simulink model "Generator_Boeing_project"  (R2019a)
settings: Solver=VariableStepAuto  StartTime=0.0  StopTime=10.0  RelTol=1e-3
values from neighbouring files (symbols this model uses):
  Lls = 4*2.822e-6    (= 1.1288e-05)    [Generator_parameters.m]
  Lmd = 4*164.571e-6    (= 0.000658284)    [Generator_parameters.m]
  Lmq = 4*125.772e-6    (= 0.000503088)    [Generator_parameters.m]
  Lpfd = 4.9*6e-6    (= 2.94e-05)    [Generator_parameters.m]
  Lpkd = 16*9.093e-6    (= 0.000145488)    [Generator_parameters.m]
  Lpkq = 16*3.175e-6    (= 5.08e-05)    [Generator_parameters.m]
  Nfds_gen = 25    [Generator_parameters.m]
  Ra = 4*2.794e-3    (= 0.011176)    [Generator_parameters.m]
  Rpfd = 4*634.998e-6    (= 0.002539992)    [Generator_parameters.m]
  Rpkd = 8*11.72e-3    (= 0.09376)    [Generator_parameters.m]
  Rpkq = 8*3.712e-3    (= 0.029696)    [Generator_parameters.m]
undefined symbols (not defined in the file or in its folder): ts
settings Model: Creator=Dominion  LastModifiedBy=Dominion

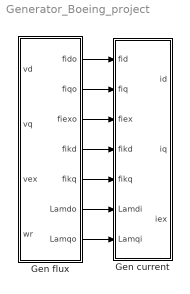
== system Generator_Boeing_project ==
  Gen current : Subsystem
  Gen flux : Subsystem
  wires:
  Gen flux/4(fikd) -> Gen current/4(fikd)
  Gen flux/5(fikq) -> Gen current/5(fikq)
  Gen flux/3(fiexo) -> Gen current/3(fiex)
  ? -> Gen flux/1(vd)
  Gen flux/7(Lamqo) -> Gen current/7(Lamqi)
  ? -> Gen flux/2(vq)
  Gen flux/2(fiqo) -> Gen current/2(fiq)
  Gen flux/6(Lamdo) -> Gen current/6(Lamdi)
  ? -> Gen flux/4(wr)
  Gen flux/1(fido) -> Gen current/1(fid)
  ? -> Gen flux/3(vex)

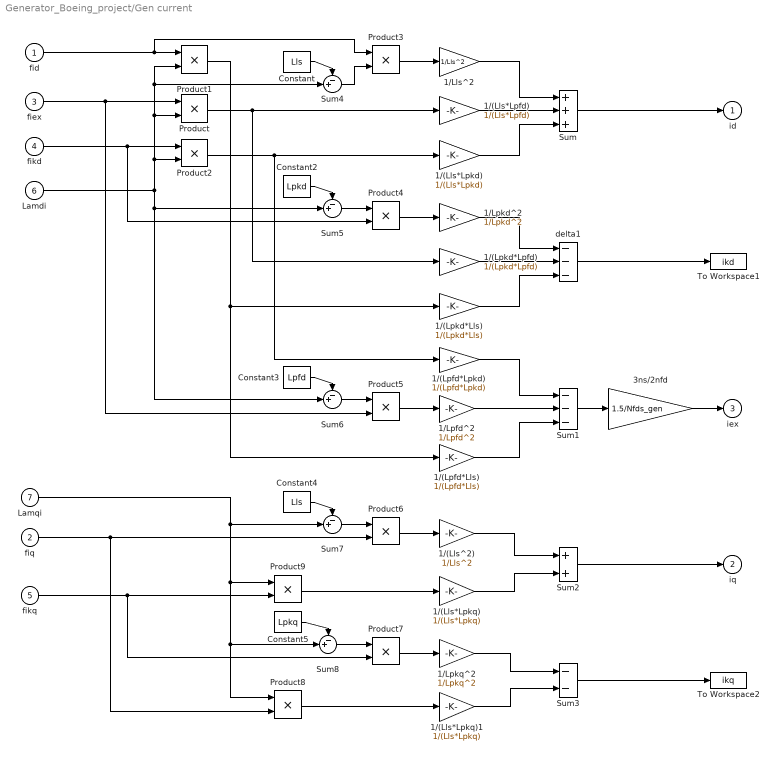
== system Generator_Boeing_project/Gen current ==
  fid : Inport
  fiq : Inport  Port=2
  fiex : Inport  Port=3
  fikd : Inport  Port=4
  fikq : Inport  Port=5
  Lamdi : Inport  Port=6
  Lamqi : Inport  Port=7
  1/(Lls*Lpfd) : Gain  Gain=1/(Lls*Lpfd)  SaturateOnIntegerOverflow=on  OutDataTypeStr=Inherit: Same as input  ParamDataTypeStr=Inherit: Same as input
  1/(Lls*Lpkd) : Gain  Gain=1/(Lls*Lpkd)  SaturateOnIntegerOverflow=on  OutDataTypeStr=Inherit: Same as input  ParamDataTypeStr=Inherit: Same as input
  1/(Lls*Lpkq) : Gain  Gain=1/(Lls*Lpkq)  SaturateOnIntegerOverflow=on  OutDataTypeStr=Inherit: Same as input  ParamDataTypeStr=Inherit: Same as input
  1/(Lls*Lpkq)1 : Gain  Gain=1/(Lls*Lpkq)  SaturateOnIntegerOverflow=on  OutDataTypeStr=Inherit: Same as input  ParamDataTypeStr=Inherit: Same as input
  1/(Lls^2) : Gain  Gain=1/Lls^2  SaturateOnIntegerOverflow=on  OutDataTypeStr=Inherit: Same as input  ParamDataTypeStr=Inherit: Same as input
  1/(Lpfd*Lls) : Gain  Gain=1/(Lpfd*Lls)  SaturateOnIntegerOverflow=on  OutDataTypeStr=Inherit: Same as input  ParamDataTypeStr=Inherit: Same as input
  1/(Lpfd*Lpkd) : Gain  Gain=1/(Lpfd*Lpkd)  SaturateOnIntegerOverflow=on  OutDataTypeStr=Inherit: Same as input  ParamDataTypeStr=Inherit: Same as input
  1/(Lpkd*Lls) : Gain  Gain=1/(Lpkd*Lls)  SaturateOnIntegerOverflow=on  OutDataTypeStr=Inherit: Same as input  ParamDataTypeStr=Inherit: Same as input
  1/(Lpkd*Lpfd) : Gain  Gain=1/(Lpkd*Lpfd)  SaturateOnIntegerOverflow=on  OutDataTypeStr=Inherit: Same as input  ParamDataTypeStr=Inherit: Same as input
  1/Lls^2 : Gain  Gain=1/Lls^2  SaturateOnIntegerOverflow=on  OutDataTypeStr=Inherit: Same as input  ParamDataTypeStr=Inherit: Same as input
  1/Lpfd^2 : Gain  Gain=1/Lpfd^2  SaturateOnIntegerOverflow=on  OutDataTypeStr=Inherit: Same as input  ParamDataTypeStr=Inherit: Same as input
  1/Lpkd^2 : Gain  Gain=1/Lpkd^2  SaturateOnIntegerOverflow=on  OutDataTypeStr=Inherit: Same as input  ParamDataTypeStr=Inherit: Same as input
  1/Lpkq^2 : Gain  Gain=1/Lpkq^2  SaturateOnIntegerOverflow=on  OutDataTypeStr=Inherit: Same as input  ParamDataTypeStr=Inherit: Same as input
  3ns/2nfd : Gain  Gain=1.5/Nfds_gen  SaturateOnIntegerOverflow=on  OutDataTypeStr=Inherit: Same as input  ParamDataTypeStr=Inherit: Same as input
  Constant : Constant  Value=Lls
  Constant2 : Constant  Value=Lpkd
  Constant3 : Constant  Value=Lpfd
  Constant4 : Constant  Value=Lls
  Constant5 : Constant  Value=Lpkq
  Product{,1..9} (10 alike) : Product  RndMeth=Zero
  Sum : Sum  Inputs=+++  SaturateOnIntegerOverflow=on  InputSameDT=on  OutDataTypeStr=Inherit: Same as first input
  Sum1 : Sum  Inputs=---  SaturateOnIntegerOverflow=on  InputSameDT=on  OutDataTypeStr=Inherit: Same as first input
  Sum2 : Sum  SaturateOnIntegerOverflow=on  InputSameDT=on  OutDataTypeStr=Inherit: Same as first input
  Sum3 : Sum  Inputs=--  SaturateOnIntegerOverflow=on  InputSameDT=on  OutDataTypeStr=Inherit: Same as first input
  Sum{4..8} (5 alike) : Sum  Inputs=-+|
  To Workspace1 : ToWorkspace  VariableName=ikd  SampleTime=ts
  To Workspace2 : ToWorkspace  VariableName=ikq  SampleTime=ts
  delta1 : Sum  Inputs=---  SaturateOnIntegerOverflow=on  InputSameDT=on  OutDataTypeStr=Inherit: Same as first input
  id : Outport
  iq : Outport  Port=2
  iex : Outport  Port=3
  wires:
  fiq/1 -> Product6/2, Product8/2
  fid/1 -> Product1/1, Product3/1
  Sum/1 -> id/1
  Sum1/1 -> 3ns/2nfd/1
  Sum2/1 -> iq/1
  1/(Lls*Lpkd)/1 -> Sum/3
  delta1/1 -> To Workspace1/1
  1/(Lpkd*Lpfd)/1 -> delta1/2
  1/Lpkd^2/1 -> delta1/1
  1/(Lpfd*Lpkd)/1 -> Sum1/1
  1/(Lls^2)/1 -> Sum2/1
  1/(Lls*Lpkq)/1 -> Sum2/2
  1/Lls^2/1 -> Sum/1
  fiex/1 -> Product/1, Product5/2
  1/(Lls*Lpfd)/1 -> Sum/2
  fikd/1 -> Product2/1, Product4/2
  1/(Lpkd*Lls)/1 -> delta1/3
  1/Lpfd^2/1 -> Sum1/2
  1/(Lpfd*Lls)/1 -> Sum1/3
  fikq/1 -> Product7/2, Product9/2
  Sum3/1 -> To Workspace2/1
  1/Lpkq^2/1 -> Sum3/1
  1/(Lls*Lpkq)1/1 -> Sum3/2
  Product/1 -> 1/(Lls*Lpfd)/1, 1/(Lpkd*Lpfd)/1
  Lamdi/1 -> Product/2, Product1/2, Sum4/2, Product2/2, Sum5/2, Sum6/2
  Product1/1 -> 1/(Lpkd*Lls)/1, 1/(Lpfd*Lls)/1
  Product2/1 -> 1/(Lls*Lpkd)/1, 1/(Lpfd*Lpkd)/1
  Product3/1 -> 1/Lls^2/1
  Constant/1 -> Sum4/1
  Sum4/1 -> Product3/2
  Product4/1 -> 1/Lpkd^2/1
  Sum5/1 -> Product4/1
  Constant2/1 -> Sum5/1
  Constant3/1 -> Sum6/1
  Product5/1 -> 1/Lpfd^2/1
  Sum6/1 -> Product5/1
  Product6/1 -> 1/(Lls^2)/1
  Lamqi/1 -> Sum7/2, Sum8/2, Product8/1, Product9/1
  Constant4/1 -> Sum7/1
  Sum7/1 -> Product6/1
  Constant5/1 -> Sum8/1
  Product7/1 -> 1/Lpkq^2/1
  Sum8/1 -> Product7/1
  Product8/1 -> 1/(Lls*Lpkq)1/1
  Product9/1 -> 1/(Lls*Lpkq)/1
  3ns/2nfd/1 -> iex/1

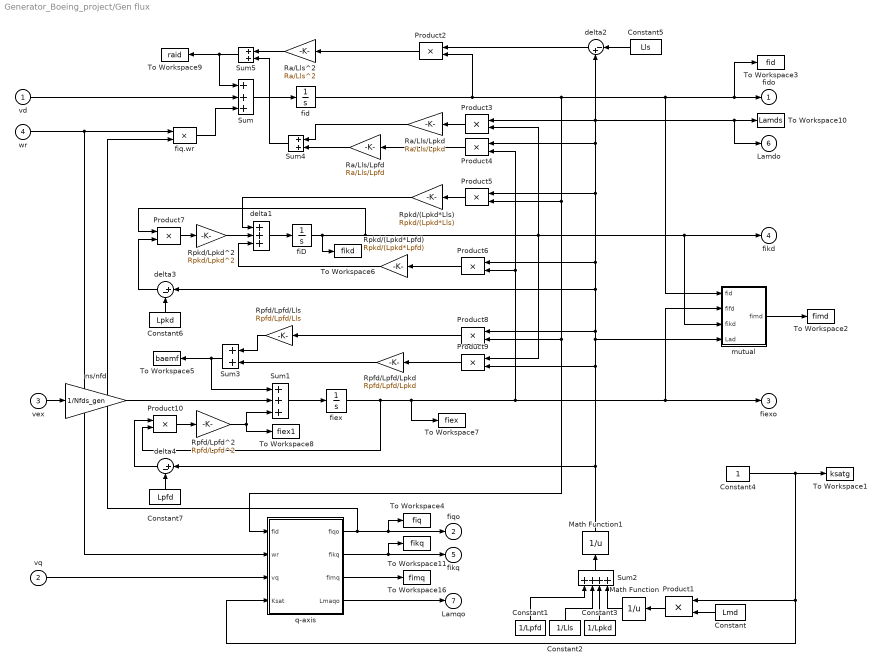
== system Generator_Boeing_project/Gen flux ==
  vd : Inport
  vq : Inport  Port=2
  vex : Inport  Port=3
  wr : Inport  Port=4
  Constant : Constant  Value=Lmd
  Constant1 : Constant  Value=1/Lpfd
  Constant2 : Constant  Value=1/Lls
  Constant3 : Constant  Value=1/Lpkd
  Constant4 : Constant
  Constant5 : Constant  Value=Lls
  Constant6 : Constant  Value=Lpkd
  Constant7 : Constant  Value=Lpfd
  Math Function : Math  Operator=reciprocal  SaturateOnIntegerOverflow=on
  Math Function1 : Math  Operator=reciprocal  SaturateOnIntegerOverflow=on
  Product{1..10} (10 alike) : Product  SaturateOnIntegerOverflow=on  OutDataTypeStr=Inherit: Same as first input
  Ra/Lls/Lpfd : Gain  Gain=Ra/Lls/Lpfd  SaturateOnIntegerOverflow=on  OutDataTypeStr=Inherit: Same as input  ParamDataTypeStr=Inherit: Same as input
  Ra/Lls/Lpkd : Gain  Gain=Ra/Lls/Lpkd  SaturateOnIntegerOverflow=on  OutDataTypeStr=Inherit: Same as input  ParamDataTypeStr=Inherit: Same as input
  Ra/Lls^2 : Gain  Gain=Ra/Lls^2  SaturateOnIntegerOverflow=on  OutDataTypeStr=Inherit: Same as input  ParamDataTypeStr=Inherit: Same as input
  Rpfd/Lpfd/Lls : Gain  Gain=Rpfd/Lpfd/Lls  SaturateOnIntegerOverflow=on  OutDataTypeStr=Inherit: Same as input  ParamDataTypeStr=Inherit: Same as input
  Rpfd/Lpfd/Lpkd : Gain  Gain=Rpfd/Lpfd/Lpkd  SaturateOnIntegerOverflow=on  OutDataTypeStr=Inherit: Same as input  ParamDataTypeStr=Inherit: Same as input
  Rpfd/Lpfd^2 : Gain  Gain=Rpfd/Lpfd^2  SaturateOnIntegerOverflow=on  OutDataTypeStr=Inherit: Same as input  ParamDataTypeStr=Inherit: Same as input
  Rpkd/(Lpkd*Lls) : Gain  Gain=Rpkd/(Lpkd*Lls)  SaturateOnIntegerOverflow=on  OutDataTypeStr=Inherit: Same as input  ParamDataTypeStr=Inherit: Same as input
  Rpkd/(Lpkd*Lpfd) : Gain  Gain=Rpkd/(Lpkd*Lpfd)  SaturateOnIntegerOverflow=on  OutDataTypeStr=Inherit: Same as input  ParamDataTypeStr=Inherit: Same as input
  Rpkd/Lpkd^2 : Gain  Gain=Rpkd/Lpkd^2  SaturateOnIntegerOverflow=on  OutDataTypeStr=Inherit: Same as input  ParamDataTypeStr=Inherit: Same as input
  Sum : Sum  Inputs=+++  SaturateOnIntegerOverflow=on  InputSameDT=on  OutDataTypeStr=Inherit: Same as first input
  Sum1 : Sum  Inputs=+++  SaturateOnIntegerOverflow=on  InputSameDT=on  OutDataTypeStr=Inherit: Same as first input
  Sum2 : Sum  Inputs=++++  SaturateOnIntegerOverflow=on  InputSameDT=on  OutDataTypeStr=Inherit: Same as first input
  Sum3 : Sum  SaturateOnIntegerOverflow=on  InputSameDT=on  OutDataTypeStr=Inherit: Same as first input
  Sum4 : Sum  SaturateOnIntegerOverflow=on  InputSameDT=on  OutDataTypeStr=Inherit: Same as first input
  Sum5 : Sum  SaturateOnIntegerOverflow=on  InputSameDT=on  OutDataTypeStr=Inherit: Same as first input
  To Workspace1 : ToWorkspace  VariableName=ksatg  SampleTime=ts
  To Workspace10 : ToWorkspace  VariableName=Lamds  SampleTime=ts
  To Workspace11 : ToWorkspace  VariableName=fikq  SampleTime=ts
  To Workspace16 : ToWorkspace  VariableName=fimq  SampleTime=ts
  To Workspace2 : ToWorkspace  VariableName=fimd  SampleTime=ts
  To Workspace3 : ToWorkspace  VariableName=fid  SampleTime=ts
  To Workspace4 : ToWorkspace  VariableName=fiq  SampleTime=ts
  To Workspace5 : ToWorkspace  VariableName=baemf  SampleTime=ts
  To Workspace6 : ToWorkspace  VariableName=fikd  SampleTime=ts
  To Workspace7 : ToWorkspace  VariableName=fiex  SampleTime=ts
  To Workspace8 : ToWorkspace  VariableName=fiex1  SampleTime=ts
  To Workspace9 : ToWorkspace  VariableName=raid  SampleTime=ts
  delta1 : Sum  Inputs=+++  SaturateOnIntegerOverflow=on  InputSameDT=on  OutDataTypeStr=Inherit: Same as first input
  delta2 : Sum  Inputs=|-+  SaturateOnIntegerOverflow=on  InputSameDT=on  OutDataTypeStr=Inherit: Same as first input
  delta3 : Sum  Inputs=|+-  SaturateOnIntegerOverflow=on  InputSameDT=on  OutDataTypeStr=Inherit: Same as first input
  delta4 : Sum  Inputs=|+-  SaturateOnIntegerOverflow=on  InputSameDT=on  OutDataTypeStr=Inherit: Same as first input
  fiD : Integrator
  fid : Integrator
  fiex : Integrator
  fiq.wr : Product  SaturateOnIntegerOverflow=on  InputSameDT=on  OutDataTypeStr=Inherit: Same as first input
  mutual : Subsystem
  ns/nfd : Gain  Gain=1/Nfds_gen  SaturateOnIntegerOverflow=on  OutDataTypeStr=Inherit: Same as input  ParamDataTypeStr=Inherit: Same as input
  q-axis : Subsystem
  fido : Outport
  fiqo : Outport  Port=2
  fiexo : Outport  Port=3
  fikd : Outport  Port=4
  fikq : Outport  Port=5
  Lamdo : Outport  Port=6
  Lamqo : Outport  Port=7
  wires:
  fid/1 -> Product5/2, q-axis/1(fid), Product8/2, mutual/1(fid), fido/1, To Workspace3/1, Product2/2
  vd/1 -> Sum/2
  Sum/1 -> fid/1
  Sum1/1 -> fiex/1
  fiq.wr/1 -> Sum/3
  fiex/1 -> Product10/2, Product4/2, Product6/2, fiexo/1, mutual/2(fifd), To Workspace7/1
  fiD/1 -> Product3/2, Product9/1, fikd/1, mutual/3(fikd), Product7/1, To Workspace6/1
  Product2/1 -> Ra/Lls^2/1
  Ra/Lls/Lpkd/1 -> Sum4/1
  Ra/Lls/Lpfd/1 -> Sum4/2
  delta1/1 -> fiD/1
  Rpkd/Lpkd^2/1 -> delta1/2
  Rpkd/(Lpkd*Lls)/1 -> delta1/1
  Rpkd/(Lpkd*Lpfd)/1 -> delta1/3
  vex/1 -> ns/nfd/1
  wr/1 -> fiq.wr/1, q-axis/2(wr)
  vq/1 -> q-axis/3(vq)
  q-axis/1(fiqo) -> fiq.wr/2, fiqo/1, To Workspace4/1
  q-axis/2(fikq) -> fikq/1, To Workspace11/1
  q-axis/3(fimq) -> To Workspace16/1
  Constant1/1 -> Sum2/1
  Constant2/1 -> Sum2/2
  Constant3/1 -> Sum2/3
  Math Function/1 -> Sum2/4
  Constant5/1 -> delta2/1
  Sum2/1 -> Math Function1/1
  delta2/1 -> Product2/1
  Product3/1 -> Ra/Lls/Lpkd/1
  Product4/1 -> Ra/Lls/Lpfd/1
  Product5/1 -> Rpkd/(Lpkd*Lls)/1
  Product6/1 -> Rpkd/(Lpkd*Lpfd)/1
  Constant6/1 -> delta3/2
  delta3/1 -> Product7/2
  Product7/1 -> Rpkd/Lpkd^2/1
  Product8/1 -> Rpfd/Lpfd/Lls/1
  Product9/1 -> Rpfd/Lpfd/Lpkd/1
  Constant7/1 -> delta4/2
  Product10/1 -> Rpfd/Lpfd^2/1
  delta4/1 -> Product10/1
  Math Function1/1 -> Product9/2, delta2/2, Product3/1, To Workspace10/1, Lamdo/1, Product4/1, Product5/1, Product6/1, delta3/1, Product8/1, mutual/4(Lad), delta4/1
  Constant/1 -> Product1/2
  Product1/1 -> Math Function/1
  mutual/1(fimd) -> To Workspace2/1
  Rpfd/Lpfd^2/1 -> Sum1/3, To Workspace8/1
  Rpfd/Lpfd/Lls/1 -> Sum3/1
  Rpfd/Lpfd/Lpkd/1 -> Sum3/2
  Sum3/1 -> Sum1/1, To Workspace5/1
  Ra/Lls^2/1 -> Sum5/1
  Sum4/1 -> Sum5/2
  Sum5/1 -> Sum/1, To Workspace9/1
  q-axis/4(Lmaqo) -> Lamqo/1
  ns/nfd/1 -> Sum1/2
  Constant4/1 -> To Workspace1/1, Product1/1, q-axis/4(Ksat)

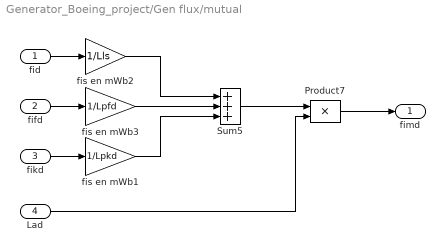
== system Generator_Boeing_project/Gen flux/mutual ==
  fid : Inport
  fifd : Inport  Port=2
  fikd : Inport  Port=3
  Lad : Inport  Port=4
  Product7 : Product  SaturateOnIntegerOverflow=on  OutDataTypeStr=Inherit: Same as first input
  Sum5 : Sum  Inputs=+++  SaturateOnIntegerOverflow=on  InputSameDT=on  OutDataTypeStr=Inherit: Same as first input
  fis en mWb1 : Gain  Gain=1/Lpkd  SaturateOnIntegerOverflow=on  OutDataTypeStr=Inherit: Same as input  ParamDataTypeStr=Inherit: Same as input
  fis en mWb2 : Gain  Gain=1/Lls  SaturateOnIntegerOverflow=on  OutDataTypeStr=Inherit: Same as input  ParamDataTypeStr=Inherit: Same as input
  fis en mWb3 : Gain  Gain=1/Lpfd  SaturateOnIntegerOverflow=on  OutDataTypeStr=Inherit: Same as input  ParamDataTypeStr=Inherit: Same as input
  fimd : Outport
  wires:
  fis en mWb1/1 -> Sum5/3
  fis en mWb3/1 -> Sum5/2
  fis en mWb2/1 -> Sum5/1
  fid/1 -> fis en mWb2/1
  fifd/1 -> fis en mWb3/1
  fikd/1 -> fis en mWb1/1
  Sum5/1 -> Product7/1
  Product7/1 -> fimd/1
  Lad/1 -> Product7/2

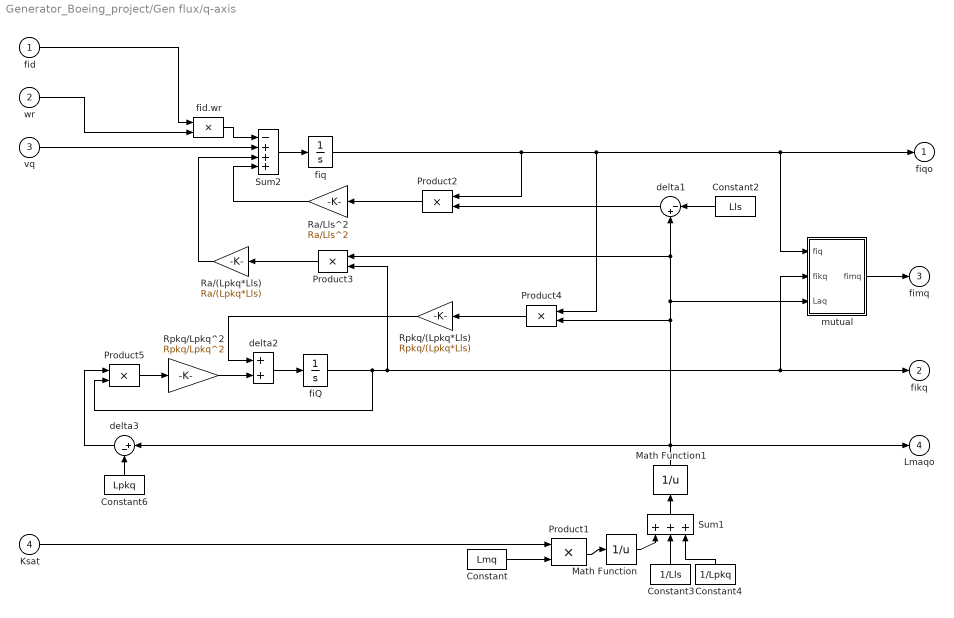
== system Generator_Boeing_project/Gen flux/q-axis ==
  fid : Inport
  wr : Inport  Port=2
  vq : Inport  Port=3
  Ksat : Inport  Port=4
  Constant : Constant  Value=Lmq
  Constant2 : Constant  Value=Lls
  Constant3 : Constant  Value=1/Lls
  Constant4 : Constant  Value=1/Lpkq
  Constant6 : Constant  Value=Lpkq
  Math Function : Math  Operator=reciprocal  SaturateOnIntegerOverflow=on
  Math Function1 : Math  Operator=reciprocal  SaturateOnIntegerOverflow=on
  Product{1..5} (5 alike) : Product  SaturateOnIntegerOverflow=on  OutDataTypeStr=Inherit: Same as first input
  Ra/(Lpkq*Lls) : Gain  Gain=Ra/(Lpkq*Lls)  SaturateOnIntegerOverflow=on  OutDataTypeStr=Inherit: Same as input  ParamDataTypeStr=Inherit: Same as input
  Ra/Lls^2 : Gain  Gain=Ra/Lls^2  SaturateOnIntegerOverflow=on  OutDataTypeStr=Inherit: Same as input  ParamDataTypeStr=Inherit: Same as input
  Rpkq/(Lpkq*Lls) : Gain  Gain=Rpkq/(Lpkq*Lls)  SaturateOnIntegerOverflow=on  OutDataTypeStr=Inherit: Same as input  ParamDataTypeStr=Inherit: Same as input
  Rpkq/Lpkq^2 : Gain  Gain=Rpkq/Lpkq^2  SaturateOnIntegerOverflow=on  OutDataTypeStr=Inherit: Same as input  ParamDataTypeStr=Inherit: Same as input
  Sum1 : Sum  Inputs=+++  SaturateOnIntegerOverflow=on  InputSameDT=on  OutDataTypeStr=Inherit: Same as first input
  Sum2 : Sum  Inputs=-+++  SaturateOnIntegerOverflow=on  InputSameDT=on  OutDataTypeStr=Inherit: Same as first input
  delta1 : Sum  Inputs=|-+  SaturateOnIntegerOverflow=on  InputSameDT=on  OutDataTypeStr=Inherit: Same as first input
  delta2 : Sum  SaturateOnIntegerOverflow=on  InputSameDT=on  OutDataTypeStr=Inherit: Same as first input
  delta3 : Sum  Inputs=|+-  SaturateOnIntegerOverflow=on  InputSameDT=on  OutDataTypeStr=Inherit: Same as first input
  fiQ : Integrator
  fid.wr : Product  SaturateOnIntegerOverflow=on  InputSameDT=on  OutDataTypeStr=Inherit: Same as first input
  fiq : Integrator
  mutual : Subsystem
  fiqo : Outport
  fikq : Outport  Port=2
  fimq : Outport  Port=3
  Lmaqo : Outport  Port=4
  wires:
  fid/1 -> fid.wr/1
  fiq/1 -> Product2/1, Product4/1, fiqo/1, mutual/1(fiq)
  vq/1 -> Sum2/2
  wr/1 -> fid.wr/2
  Sum2/1 -> fiq/1
  fid.wr/1 -> Sum2/1
  Ra/Lls^2/1 -> Sum2/4
  Ra/(Lpkq*Lls)/1 -> Sum2/3
  fiQ/1 -> Product3/2, fikq/1, mutual/2(fikq), Product5/2
  Rpkq/Lpkq^2/1 -> delta2/2
  delta2/1 -> fiQ/1
  Rpkq/(Lpkq*Lls)/1 -> delta2/1
  Constant/1 -> Product1/2
  Product1/1 -> Math Function/1
  Math Function/1 -> Sum1/1
  Constant4/1 -> Sum1/3
  Ksat/1 -> Product1/1
  Constant3/1 -> Sum1/2
  Constant2/1 -> delta1/1
  Sum1/1 -> Math Function1/1
  Product2/1 -> Ra/Lls^2/1
  delta1/1 -> Product2/2
  Product3/1 -> Ra/(Lpkq*Lls)/1
  Product4/1 -> Rpkq/(Lpkq*Lls)/1
  Constant6/1 -> delta3/2
  Product5/1 -> Rpkq/Lpkq^2/1
  delta3/1 -> Product5/1
  Math Function1/1 -> Product4/2, delta1/2, Product3/1, mutual/3(Laq), delta3/1, Lmaqo/1
  mutual/1(fimq) -> fimq/1

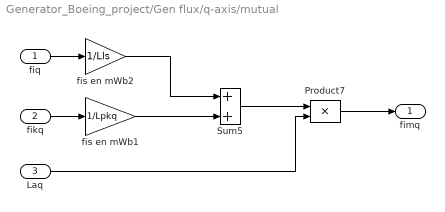
== system Generator_Boeing_project/Gen flux/q-axis/mutual ==
  fiq : Inport
  fikq : Inport  Port=2
  Laq : Inport  Port=3
  Product7 : Product  SaturateOnIntegerOverflow=on  OutDataTypeStr=Inherit: Same as first input
  Sum5 : Sum  SaturateOnIntegerOverflow=on  InputSameDT=on  OutDataTypeStr=Inherit: Same as first input
  fis en mWb1 : Gain  Gain=1/Lpkq  SaturateOnIntegerOverflow=on  OutDataTypeStr=Inherit: Same as input  ParamDataTypeStr=Inherit: Same as input
  fis en mWb2 : Gain  Gain=1/Lls  SaturateOnIntegerOverflow=on  OutDataTypeStr=Inherit: Same as input  ParamDataTypeStr=Inherit: Same as input
  fimq : Outport
  wires:
  fis en mWb1/1 -> Sum5/2
  fis en mWb2/1 -> Sum5/1
  fiq/1 -> fis en mWb2/1
  fikq/1 -> fis en mWb1/1
  Sum5/1 -> Product7/1
  Product7/1 -> fimq/1
  Laq/1 -> Product7/2
